simulink model "SistemaCAS_v20"  (R2014a)
settings: Solver=ode3  StartTime=0.0  StopTime=0.009  FixedStep=0.000001  RelTol=1e-3
libraries: simulink x21, dspmathops x10, commchan3 x1
settings Model: Creator=andre  LastModifiedBy=andre
settings DebuggingCC: SolverPrmCheckMsg=none

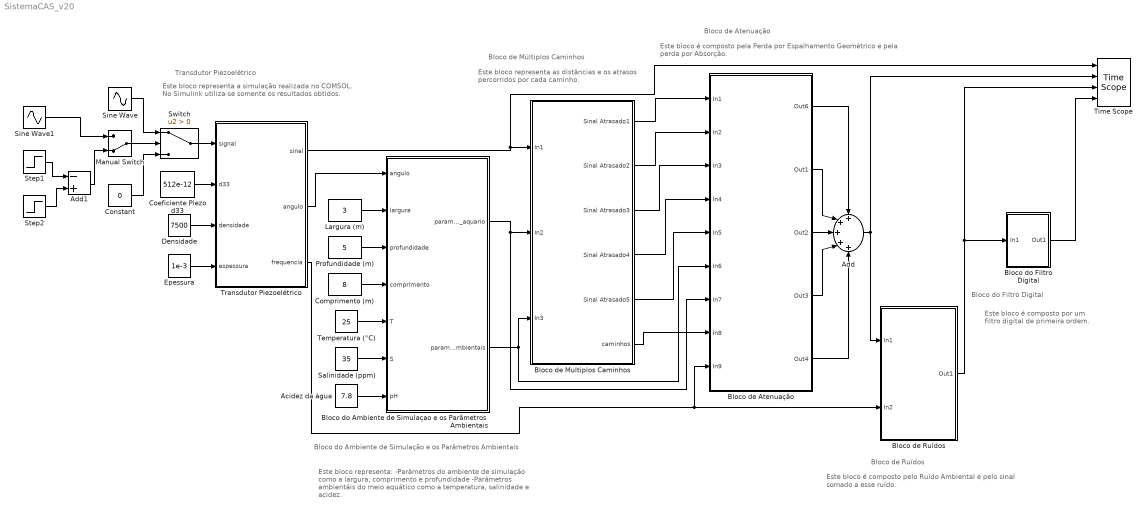
== system SistemaCAS_v20 ==
  note: Este bloco representa a simulação realizada no COMSOL. No Simulink utiliza-se somente os resultados obtidos.
  note: Transdutor Piezoelétrico
  note: Este bloco representa:
      | -Parâmetros do ambiente de simulação como a largura, comprimento e profundidade
      | -Parâmetros ambientáis do meio aquático como a temperatura, salinidade e acidez.
  note: Bloco do Ambiente de Simulação e os Parâmetros Ambientais
  note: Este bloco representa as distâncias e
      | os atrasos percorridos por cada caminho.
  note: Bloco de Múltiplos Caminhos
  note: Este bloco é composto pela Perda por Espalhamento Geométrico e pela perda por Absorção.
  note: Bloco de Atenuação
  note: Este bloco é composto pelo Ruído Ambiental e pelo sinal somado a esse ruído.
  note: Bloco de Ruídos
  note: Este bloco é composto
      | por um filtro digital
      | de primeira ordem.
  note: Bloco do Filtro Digital
  Acidez da água : Constant  Value=7.8
  Add : Sum  Inputs=+++++
  Add1 : Sum  Inputs=-+
  Bloco de Atenuação : Subsystem
  Bloco de Multiplos Caminhos : Subsystem
  Bloco de Ruídos : Subsystem
  Bloco do Ambiente de Simulaçao e os Parâmetros Ambientais : MATLAB Function  TreatAsAtomicUnit=on
  Bloco do Filtro Digital : Subsystem
  Coeficiente Piezo d33 : Constant  Value=512e-12
  Comprimento (m) : Constant  Value=8
  Constant : Constant  Value=0
  Densidade : Constant  Value=7500
  Epessura : Constant  Value=1e-3
  Largura (m) : Constant  Value=3
  Manual Switch : ManualSwitch  CurrentSetting=0
  Profundidade (m) : Constant  Value=5
  Salinidade (ppm) : Constant  Value=35
  Sine Wave : Sin  Amplitude=10  Frequency=19670*(2*pi)  Samples=51  SampleTime=1/1000000
  Sine Wave1 : Sin  Amplitude=10  Frequency=2000*(2*pi)  Samples=100  SampleTime=1/1000000
  Step1 : Step  Time=5*(1/19670)  SampleTime=1/1000000
  Step2 : Step  Time=0  SampleTime=1/1000000
  Switch : Switch  Criteria=u2 > Threshold
  Temperatura (°C) : Constant  Value=25
  Time Scope : TimeScope  NumInputPorts=4  DefaultConfigurationName=spbscopes.TimeScopeBlockCfg
  Transdutor Piezoelétrico : MATLAB Function  TreatAsAtomicUnit=on
  wires:
  Sine Wave/1 -> Switch/1
  Constant/1 -> Switch/3
  Largura (m)/1 -> Bloco do Ambiente de Simulaçao e os Parâmetros Ambientais/2(largura)
  Profundidade (m)/1 -> Bloco do Ambiente de Simulaçao e os Parâmetros Ambientais/3(profundidade)
  Coeficiente Piezo d33/1 -> Transdutor Piezoelétrico/2(d33)
  Densidade/1 -> Transdutor Piezoelétrico/3(densidade)
  Epessura/1 -> Transdutor Piezoelétrico/4(espessura)
  Transdutor Piezoelétrico/2(angulo) -> Bloco do Ambiente de Simulaçao e os Parâmetros Ambientais/1(angulo)
  Bloco do Ambiente de Simulaçao e os Parâmetros Ambientais/1(parametros_aquario) -> Bloco de Atenuação/7(In7), Bloco de Multiplos Caminhos/2(In2)
  Bloco do Ambiente de Simulaçao e os Parâmetros Ambientais/2(parametros_ambientais) -> Bloco de Multiplos Caminhos/3(In3), Bloco de Atenuação/6(In6)
  Switch/1 -> Transdutor Piezoelétrico/1(signal)
  Transdutor Piezoelétrico/3(frequencia) -> Bloco de Ruídos/2(In2), Bloco de Atenuação/9(In9)
  Temperatura (°C)/1 -> Bloco do Ambiente de Simulaçao e os Parâmetros Ambientais/5(T)
  Salinidade (ppm)/1 -> Bloco do Ambiente de Simulaçao e os Parâmetros Ambientais/6(S)
  Acidez da água/1 -> Bloco do Ambiente de Simulaçao e os Parâmetros Ambientais/7(pH)
  Bloco de Multiplos Caminhos/1(Sinal Atrasado1) -> Bloco de Atenuação/1(In1)
  Bloco de Multiplos Caminhos/2(Sinal Atrasado2) -> Bloco de Atenuação/2(In2)
  Bloco de Multiplos Caminhos/3(Sinal Atrasado3) -> Bloco de Atenuação/3(In3)
  Bloco de Multiplos Caminhos/5(Sinal Atrasado5) -> Bloco de Atenuação/5(In5)
  Bloco de Multiplos Caminhos/6(caminhos) -> Bloco de Atenuação/8(In8)
  Bloco de Multiplos Caminhos/4(Sinal Atrasado4) -> Bloco de Atenuação/4(In4)
  Add/1 -> Bloco de Ruídos/1(In1), Time Scope/2
  Bloco de Atenuação/1(Out6) -> Add/1
  Bloco de Atenuação/2(Out1) -> Add/2
  Bloco de Atenuação/3(Out2) -> Add/3
  Bloco de Atenuação/4(Out3) -> Add/4
  Bloco de Atenuação/5(Out4) -> Add/5
  Comprimento (m)/1 -> Bloco do Ambiente de Simulaçao e os Parâmetros Ambientais/4(comprimento)
  Bloco de Ruídos/1(Out1) -> Time Scope/3, Bloco do Filtro Digital/1(In1)
  Step1/1 -> Add1/1
  Step2/1 -> Add1/2
  Manual Switch/1 -> Switch/2
  Sine Wave1/1 -> Manual Switch/1
  Add1/1 -> Manual Switch/2
  Transdutor Piezoelétrico/1(sinal) -> Time Scope/1, Bloco de Multiplos Caminhos/1(In1)
  Bloco do Filtro Digital/1(Out1) -> Time Scope/4

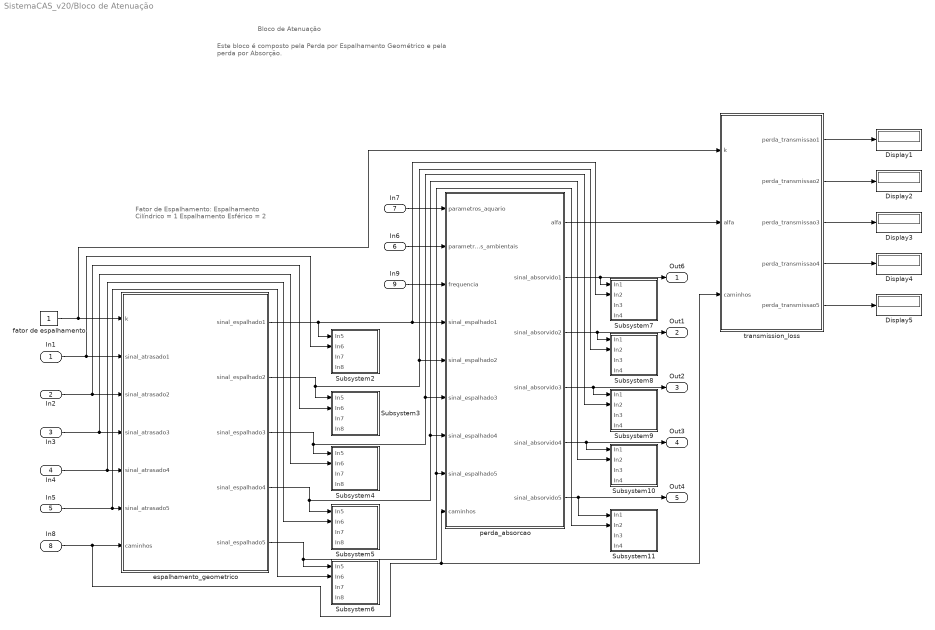
== system SistemaCAS_v20/Bloco de Atenuação ==
  note: Fator de Espalhamento:
      |
      | Espalhamento Cilíndrico = 1
      | Espalhamento Esférico = 2
  note: Este bloco é composto pela Perda por Espalhamento Geométrico e pela perda por Absorção.
  note: Bloco de Atenuação
  In1 : Inport
  In2 : Inport  Port=2
  In3 : Inport  Port=3
  In4 : Inport  Port=4
  In5 : Inport  Port=5
  In6 : Inport  Port=6
  In7 : Inport  Port=7
  In8 : Inport  Port=8
  In9 : Inport  Port=9
  Display{1..5} (5 alike) : Display
      settings: Decimation=2
  Subsystem10 : Subsystem
  Subsystem11 : Subsystem
  Subsystem2 : Subsystem
  Subsystem3 : Subsystem
  Subsystem4 : Subsystem
  Subsystem5 : Subsystem
  Subsystem6 : Subsystem
  Subsystem7 : Subsystem
  Subsystem8 : Subsystem
  Subsystem9 : Subsystem
  espalhamento_geometrico : MATLAB Function  TreatAsAtomicUnit=on
  fator de espalhamento : Constant
  perda_absorcao : MATLAB Function  TreatAsAtomicUnit=on
  transmission_loss : MATLAB Function  TreatAsAtomicUnit=on
  Out6 : Outport
  Out1 : Outport  Port=2
  Out2 : Outport  Port=3
  Out3 : Outport  Port=4
  Out4 : Outport  Port=5
  wires:
  espalhamento_geometrico/1(sinal_espalhado1) -> Subsystem2/1(In5), perda_absorcao/4(sinal_espalhado1), Subsystem7/2(In2)
  In1/1 -> Subsystem2/2(In6), espalhamento_geometrico/2(sinal_atrasado1)
  In3/1 -> Subsystem4/2(In6), espalhamento_geometrico/4(sinal_atrasado3)
  In4/1 -> Subsystem5/2(In6), espalhamento_geometrico/5(sinal_atrasado4)
  fator de espalhamento/1 -> transmission_loss/1(k), espalhamento_geometrico/1(k)
  espalhamento_geometrico/2(sinal_espalhado2) -> Subsystem3/1(In5), perda_absorcao/5(sinal_espalhado2), Subsystem8/2(In2)
  espalhamento_geometrico/5(sinal_espalhado5) -> Subsystem6/1(In5), Subsystem11/2(In2), perda_absorcao/8(sinal_espalhado5)
  espalhamento_geometrico/3(sinal_espalhado3) -> Subsystem4/1(In5), perda_absorcao/6(sinal_espalhado3), Subsystem9/2(In2)
  espalhamento_geometrico/4(sinal_espalhado4) -> Subsystem5/1(In5), perda_absorcao/7(sinal_espalhado4), Subsystem10/2(In2)
  In6/1 -> perda_absorcao/2(parametros_ambientais)
  In7/1 -> perda_absorcao/1(parametros_aquario)
  In9/1 -> perda_absorcao/3(frequencia)
  perda_absorcao/2(sinal_absorvido1) -> Subsystem7/1(In1), Out6/1
  perda_absorcao/5(sinal_absorvido4) -> Out3/1, Subsystem10/1(In1)
  perda_absorcao/6(sinal_absorvido5) -> Out4/1, Subsystem11/1(In1)
  transmission_loss/1(perda_transmissao1) -> Display1/1
  In2/1 -> Subsystem3/2(In6), espalhamento_geometrico/3(sinal_atrasado2)
  perda_absorcao/4(sinal_absorvido3) -> Out2/1, Subsystem9/1(In1)
  perda_absorcao/1(alfa) -> transmission_loss/2(alfa)
  perda_absorcao/3(sinal_absorvido2) -> Out1/1, Subsystem8/1(In1)
  In5/1 -> Subsystem6/2(In6), espalhamento_geometrico/6(sinal_atrasado5)
  In8/1 -> perda_absorcao/9(caminhos), transmission_loss/3(caminhos), espalhamento_geometrico/7(caminhos)
  transmission_loss/2(perda_transmissao2) -> Display2/1
  transmission_loss/3(perda_transmissao3) -> Display3/1
  transmission_loss/4(perda_transmissao4) -> Display4/1
  transmission_loss/5(perda_transmissao5) -> Display5/1

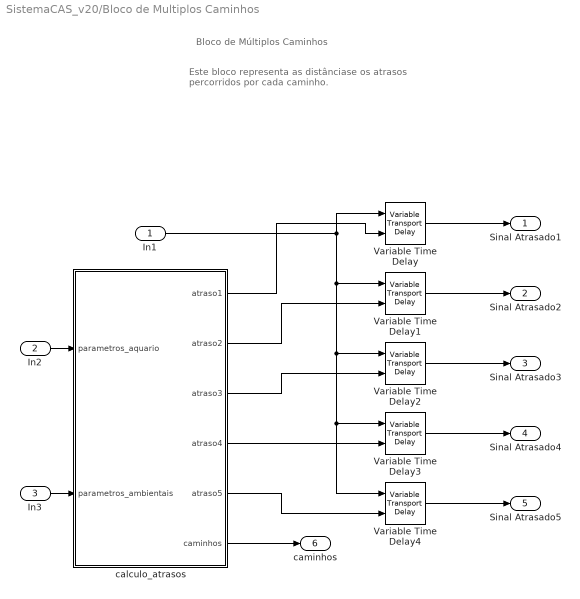
== system SistemaCAS_v20/Bloco de Multiplos Caminhos ==
  note: Este bloco representa as distânciase os atrasos percorridos por cada caminho.
  note: Bloco de Múltiplos Caminhos
  In1 : Inport
  In2 : Inport  Port=2
  In3 : Inport  Port=3
  Variable Time Delay{,1..4} (5 alike) : VariableTransportDelay  MaximumDelay=10
  calculo_atrasos : MATLAB Function  TreatAsAtomicUnit=on
  Sinal Atrasado1 : Outport
  Sinal Atrasado2 : Outport  Port=2
  Sinal Atrasado3 : Outport  Port=3
  Sinal Atrasado4 : Outport  Port=4
  Sinal Atrasado5 : Outport  Port=5
  caminhos : Outport  Port=6
  wires:
  calculo_atrasos/3(atraso3) -> Variable Time Delay2/2
  In2/1 -> calculo_atrasos/1(parametros_aquario)
  In3/1 -> calculo_atrasos/2(parametros_ambientais)
  In1/1 -> Variable Time Delay/1, Variable Time Delay1/1, Variable Time Delay2/1, Variable Time Delay4/1, Variable Time Delay3/1
  calculo_atrasos/1(atraso1) -> Variable Time Delay/2
  Variable Time Delay1/1 -> Sinal Atrasado2/1
  Variable Time Delay3/1 -> Sinal Atrasado4/1
  Variable Time Delay2/1 -> Sinal Atrasado3/1
  calculo_atrasos/6(caminhos) -> caminhos/1
  calculo_atrasos/2(atraso2) -> Variable Time Delay1/2
  calculo_atrasos/4(atraso4) -> Variable Time Delay3/2
  calculo_atrasos/5(atraso5) -> Variable Time Delay4/2
  Variable Time Delay/1 -> Sinal Atrasado1/1
  Variable Time Delay4/1 -> Sinal Atrasado5/1

== system SistemaCAS_v20/Bloco de Ruídos ==
  note: Este bloco é composto pelo Ruído Ambiental e pelo sinal somado a esse ruído.
  note: Bloco de Ruídos
  In1 : Inport
  In2 : Inport  Port=2
  AWGN Channel : commchan3/AWGN Channel  InputProcessing=Columns as channels (frame based)  seed=1  noiseMode=Variance from port  EbNodB=10  EsNodB=10  SNRdB=0  bitsPerSym=1  Ps=1  Tsym=1  variance=1
  To Workspace : ToWorkspace  VariableName=semruido  SaveFormat=Timeseries  SampleTime=-1
  To Workspace1 : ToWorkspace  VariableName=comruido  SaveFormat=Timeseries  SampleTime=-1
  fator de navegação (0-1) : Constant  Value=0
  ruido_ambiente : MATLAB Function  TreatAsAtomicUnit=on
  velocidade do vento (m/s) : Constant  Value=4.17
  Out1 : Outport
  wires:
  In2/1 -> ruido_ambiente/1(frequencia)
  AWGN Channel/1 -> Out1/1, To Workspace1/1
  fator de navegação (0-1)/1 -> ruido_ambiente/2(n)
  velocidade do vento (m/s)/1 -> ruido_ambiente/3(v)
  In1/1 -> To Workspace/1, AWGN Channel/1
  ruido_ambiente/1(ruido_total) -> AWGN Channel/2

== system SistemaCAS_v20/Bloco do Filtro Digital ==
  In1 : Inport
  Transfer Fcn First Order : simulink/Discrete/Transfer Fcn First Order  PoleZ=0.93  ICPrevOutput=0.0  RndMeth=Round  DoSatur=off
  Out1 : Outport
  wires:
  Transfer Fcn First Order/1 -> Out1/1
  In1/1 -> Transfer Fcn First Order/1

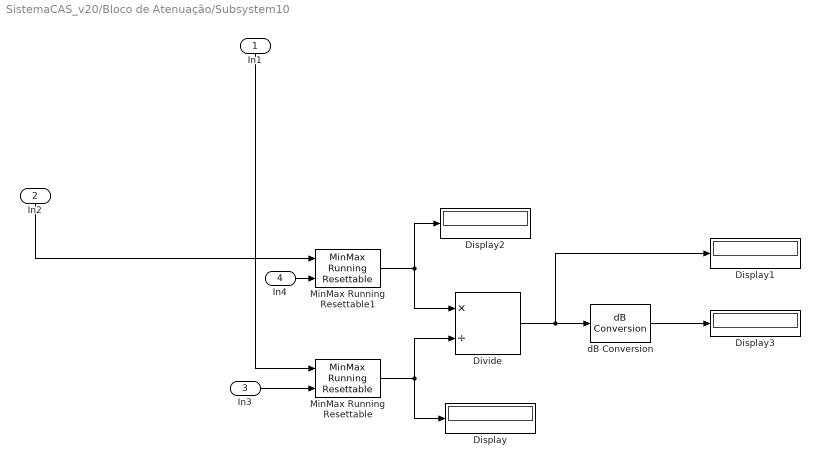
== system SistemaCAS_v20/Bloco de Atenuação/Subsystem10 ==
  In1 : Inport
  In2 : Inport  Port=2
  In3 : Inport  Port=3
  In4 : Inport  Port=4
  Display{,1..3} (4 alike) : Display
      Display1 settings: Decimation=2
      Display3 settings: Decimation=2
  Divide : Product  Inputs=*/
  MinMax Running Resettable : simulink/Math Operations/MinMax Running Resettable  Function=max  vinit=0.0
  MinMax Running Resettable1 : simulink/Math Operations/MinMax Running Resettable  Function=max  vinit=0.0
  dB Conversion : dspmathops/dB Conversion  dBtype=dB  intype=Power  R=1  fuzz=off
  wires:
  In4/1 -> MinMax Running Resettable1/2
  In1/1 -> MinMax Running Resettable/1
  In3/1 -> MinMax Running Resettable/2
  dB Conversion/1 -> Display3/1
  MinMax Running Resettable1/1 -> Display2/1, Divide/1
  MinMax Running Resettable/1 -> Display/1, Divide/2
  Divide/1 -> dB Conversion/1, Display1/1
  In2/1 -> MinMax Running Resettable1/1

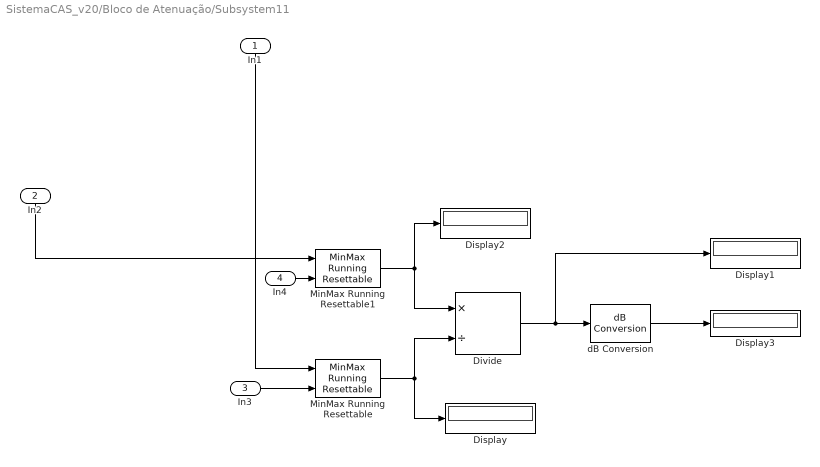
== system SistemaCAS_v20/Bloco de Atenuação/Subsystem11 ==
  In1 : Inport
  In2 : Inport  Port=2
  In3 : Inport  Port=3
  In4 : Inport  Port=4
  Display{,1..3} (4 alike) : Display
      Display1 settings: Decimation=2
      Display3 settings: Decimation=2
  Divide : Product  Inputs=*/
  MinMax Running Resettable : simulink/Math Operations/MinMax Running Resettable  Function=max  vinit=0.0
  MinMax Running Resettable1 : simulink/Math Operations/MinMax Running Resettable  Function=max  vinit=0.0
  dB Conversion : dspmathops/dB Conversion  dBtype=dB  intype=Power  R=1  fuzz=off
  wires:
  In4/1 -> MinMax Running Resettable1/2
  In1/1 -> MinMax Running Resettable/1
  In3/1 -> MinMax Running Resettable/2
  dB Conversion/1 -> Display3/1
  MinMax Running Resettable1/1 -> Display2/1, Divide/1
  MinMax Running Resettable/1 -> Display/1, Divide/2
  Divide/1 -> dB Conversion/1, Display1/1
  In2/1 -> MinMax Running Resettable1/1

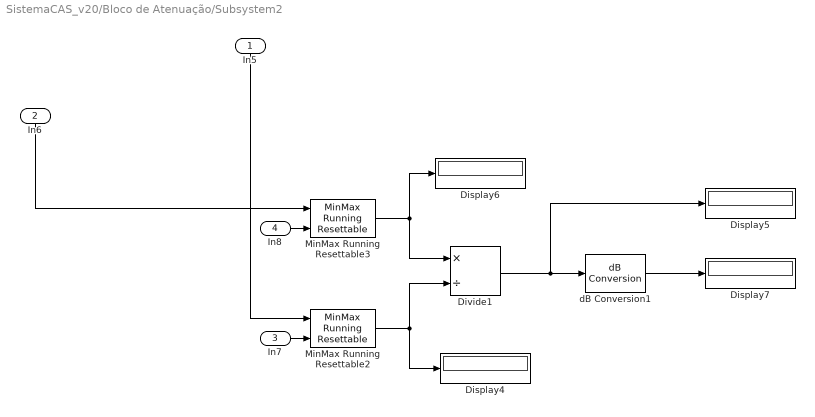
== system SistemaCAS_v20/Bloco de Atenuação/Subsystem2 ==
  In5 : Inport
  In6 : Inport  Port=2
  In7 : Inport  Port=3
  In8 : Inport  Port=4
  Display{4..7} (4 alike) : Display
      Display5 settings: Decimation=2
      Display7 settings: Decimation=2
  Divide1 : Product  Inputs=*/
  MinMax Running Resettable2 : simulink/Math Operations/MinMax Running Resettable  Function=max  vinit=0.0
  MinMax Running Resettable3 : simulink/Math Operations/MinMax Running Resettable  Function=max  vinit=0.0
  dB Conversion1 : dspmathops/dB Conversion  dBtype=dB  intype=Power  R=1  fuzz=off
  wires:
  In8/1 -> MinMax Running Resettable3/2
  In6/1 -> MinMax Running Resettable3/1
  In5/1 -> MinMax Running Resettable2/1
  In7/1 -> MinMax Running Resettable2/2
  dB Conversion1/1 -> Display7/1
  MinMax Running Resettable3/1 -> Display6/1, Divide1/1
  MinMax Running Resettable2/1 -> Display4/1, Divide1/2
  Divide1/1 -> dB Conversion1/1, Display5/1

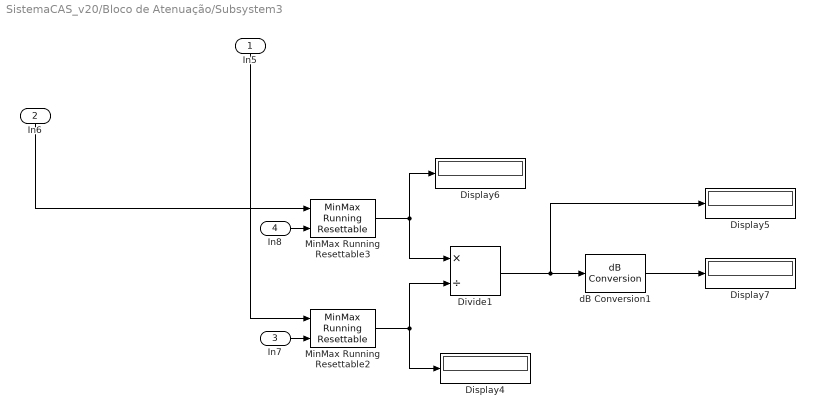
== system SistemaCAS_v20/Bloco de Atenuação/Subsystem3 ==
  In5 : Inport
  In6 : Inport  Port=2
  In7 : Inport  Port=3
  In8 : Inport  Port=4
  Display{4..7} (4 alike) : Display
      Display5 settings: Decimation=2
      Display7 settings: Decimation=2
  Divide1 : Product  Inputs=*/
  MinMax Running Resettable2 : simulink/Math Operations/MinMax Running Resettable  Function=max  vinit=0.0
  MinMax Running Resettable3 : simulink/Math Operations/MinMax Running Resettable  Function=max  vinit=0.0
  dB Conversion1 : dspmathops/dB Conversion  dBtype=dB  intype=Power  R=1  fuzz=off
  wires:
  In8/1 -> MinMax Running Resettable3/2
  In6/1 -> MinMax Running Resettable3/1
  In5/1 -> MinMax Running Resettable2/1
  In7/1 -> MinMax Running Resettable2/2
  dB Conversion1/1 -> Display7/1
  MinMax Running Resettable3/1 -> Display6/1, Divide1/1
  MinMax Running Resettable2/1 -> Display4/1, Divide1/2
  Divide1/1 -> dB Conversion1/1, Display5/1

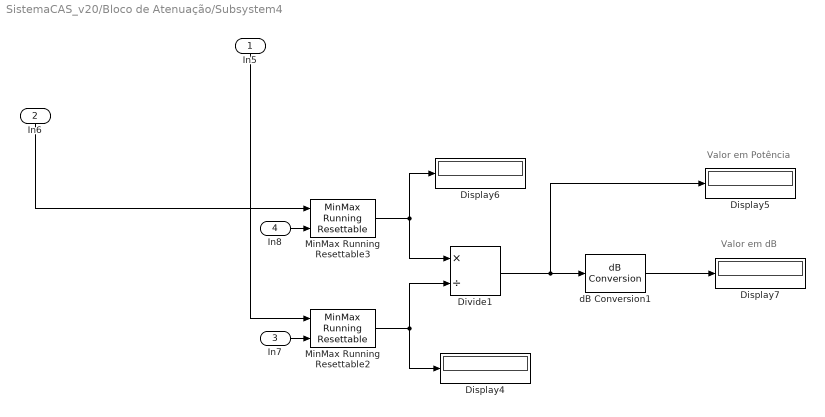
== system SistemaCAS_v20/Bloco de Atenuação/Subsystem4 ==
  note: Valor em dB
  note: Valor em Potência
  In5 : Inport
  In6 : Inport  Port=2
  In7 : Inport  Port=3
  In8 : Inport  Port=4
  Display{4..7} (4 alike) : Display
      Display5 settings: Decimation=2
      Display7 settings: Decimation=2
  Divide1 : Product  Inputs=*/
  MinMax Running Resettable2 : simulink/Math Operations/MinMax Running Resettable  Function=max  vinit=0.0
  MinMax Running Resettable3 : simulink/Math Operations/MinMax Running Resettable  Function=max  vinit=0.0
  dB Conversion1 : dspmathops/dB Conversion  dBtype=dB  intype=Power  R=1  fuzz=off
  wires:
  In8/1 -> MinMax Running Resettable3/2
  In6/1 -> MinMax Running Resettable3/1
  In5/1 -> MinMax Running Resettable2/1
  In7/1 -> MinMax Running Resettable2/2
  dB Conversion1/1 -> Display7/1
  MinMax Running Resettable3/1 -> Display6/1, Divide1/1
  MinMax Running Resettable2/1 -> Display4/1, Divide1/2
  Divide1/1 -> dB Conversion1/1, Display5/1

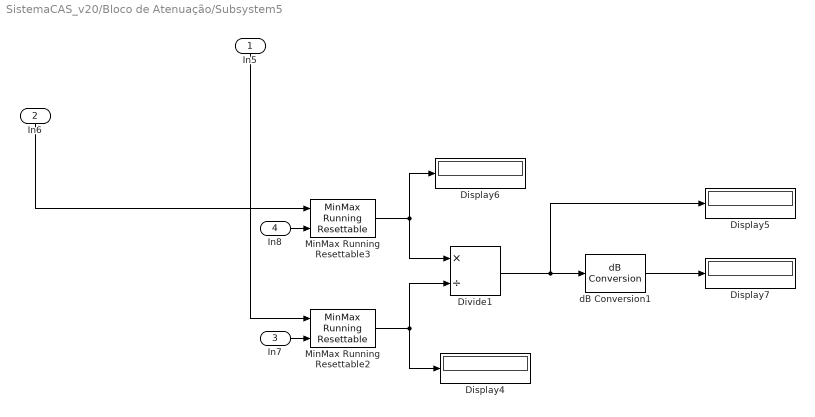
== system SistemaCAS_v20/Bloco de Atenuação/Subsystem5 ==
  In5 : Inport
  In6 : Inport  Port=2
  In7 : Inport  Port=3
  In8 : Inport  Port=4
  Display{4..7} (4 alike) : Display
      Display5 settings: Decimation=2
      Display7 settings: Decimation=2
  Divide1 : Product  Inputs=*/
  MinMax Running Resettable2 : simulink/Math Operations/MinMax Running Resettable  Function=max  vinit=0.0
  MinMax Running Resettable3 : simulink/Math Operations/MinMax Running Resettable  Function=max  vinit=0.0
  dB Conversion1 : dspmathops/dB Conversion  dBtype=dB  intype=Power  R=1  fuzz=off
  wires:
  In8/1 -> MinMax Running Resettable3/2
  In6/1 -> MinMax Running Resettable3/1
  In5/1 -> MinMax Running Resettable2/1
  In7/1 -> MinMax Running Resettable2/2
  dB Conversion1/1 -> Display7/1
  MinMax Running Resettable3/1 -> Display6/1, Divide1/1
  MinMax Running Resettable2/1 -> Display4/1, Divide1/2
  Divide1/1 -> dB Conversion1/1, Display5/1

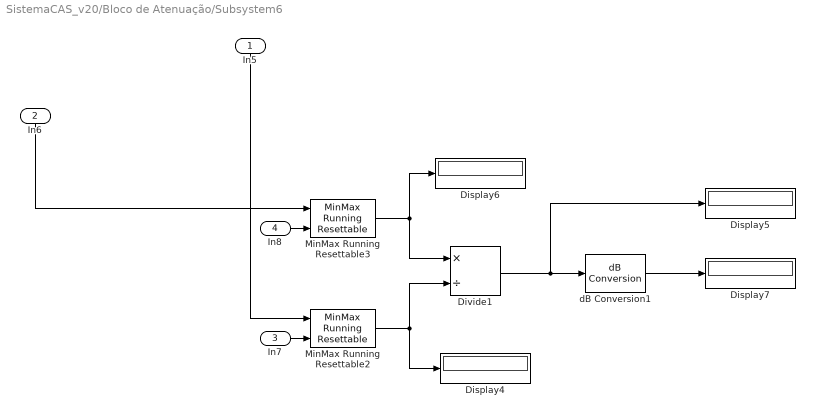
== system SistemaCAS_v20/Bloco de Atenuação/Subsystem6 ==
  In5 : Inport
  In6 : Inport  Port=2
  In7 : Inport  Port=3
  In8 : Inport  Port=4
  Display{4..7} (4 alike) : Display
      Display5 settings: Decimation=2
      Display7 settings: Decimation=2
  Divide1 : Product  Inputs=*/
  MinMax Running Resettable2 : simulink/Math Operations/MinMax Running Resettable  Function=max  vinit=0.0
  MinMax Running Resettable3 : simulink/Math Operations/MinMax Running Resettable  Function=max  vinit=0.0
  dB Conversion1 : dspmathops/dB Conversion  dBtype=dB  intype=Power  R=1  fuzz=off
  wires:
  In8/1 -> MinMax Running Resettable3/2
  In6/1 -> MinMax Running Resettable3/1
  In5/1 -> MinMax Running Resettable2/1
  In7/1 -> MinMax Running Resettable2/2
  dB Conversion1/1 -> Display7/1
  MinMax Running Resettable3/1 -> Display6/1, Divide1/1
  MinMax Running Resettable2/1 -> Display4/1, Divide1/2
  Divide1/1 -> dB Conversion1/1, Display5/1

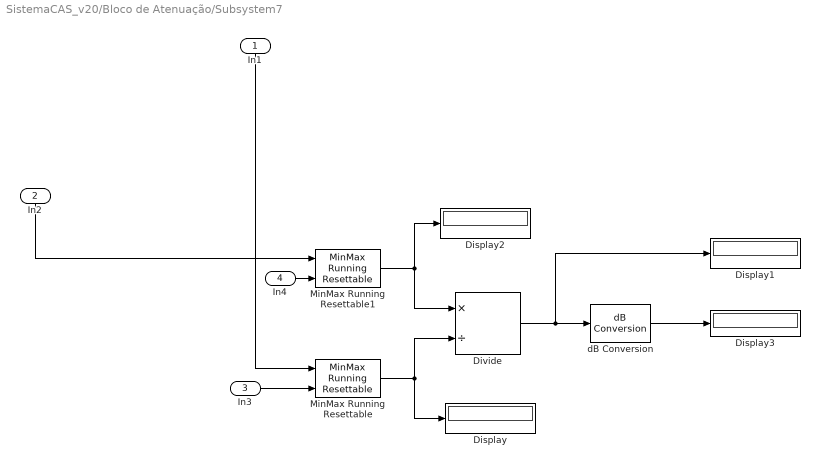
== system SistemaCAS_v20/Bloco de Atenuação/Subsystem7 ==
  In1 : Inport
  In2 : Inport  Port=2
  In3 : Inport  Port=3
  In4 : Inport  Port=4
  Display{,1..3} (4 alike) : Display
      Display1 settings: Decimation=2
      Display3 settings: Decimation=2
  Divide : Product  Inputs=*/
  MinMax Running Resettable : simulink/Math Operations/MinMax Running Resettable  Function=max  vinit=0.0
  MinMax Running Resettable1 : simulink/Math Operations/MinMax Running Resettable  Function=max  vinit=0.0
  dB Conversion : dspmathops/dB Conversion  dBtype=dB  intype=Power  R=1  fuzz=off
  wires:
  In4/1 -> MinMax Running Resettable1/2
  In1/1 -> MinMax Running Resettable/1
  In3/1 -> MinMax Running Resettable/2
  dB Conversion/1 -> Display3/1
  MinMax Running Resettable1/1 -> Display2/1, Divide/1
  MinMax Running Resettable/1 -> Display/1, Divide/2
  Divide/1 -> dB Conversion/1, Display1/1
  In2/1 -> MinMax Running Resettable1/1

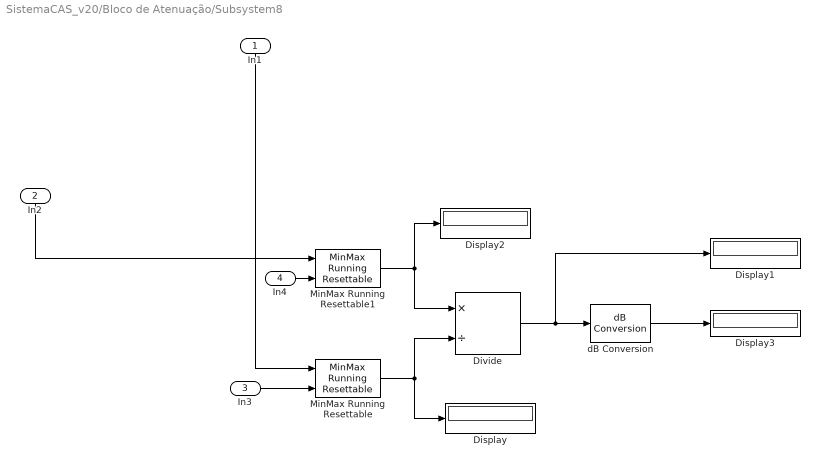
== system SistemaCAS_v20/Bloco de Atenuação/Subsystem8 ==
  In1 : Inport
  In2 : Inport  Port=2
  In3 : Inport  Port=3
  In4 : Inport  Port=4
  Display{,1..3} (4 alike) : Display
      Display1 settings: Decimation=2
      Display3 settings: Decimation=2
  Divide : Product  Inputs=*/
  MinMax Running Resettable : simulink/Math Operations/MinMax Running Resettable  Function=max  vinit=0.0
  MinMax Running Resettable1 : simulink/Math Operations/MinMax Running Resettable  Function=max  vinit=0.0
  dB Conversion : dspmathops/dB Conversion  dBtype=dB  intype=Power  R=1  fuzz=off
  wires:
  In4/1 -> MinMax Running Resettable1/2
  In1/1 -> MinMax Running Resettable/1
  In3/1 -> MinMax Running Resettable/2
  dB Conversion/1 -> Display3/1
  MinMax Running Resettable1/1 -> Display2/1, Divide/1
  MinMax Running Resettable/1 -> Display/1, Divide/2
  Divide/1 -> dB Conversion/1, Display1/1
  In2/1 -> MinMax Running Resettable1/1

== system SistemaCAS_v20/Bloco de Atenuação/Subsystem9 ==
  note: Valor em dB
  note: Valor em Potência
  In1 : Inport
  In2 : Inport  Port=2
  In3 : Inport  Port=3
  In4 : Inport  Port=4
  Display{,1..3} (4 alike) : Display
      Display1 settings: Decimation=2
      Display3 settings: Decimation=2
  Divide : Product  Inputs=*/
  MinMax Running Resettable : simulink/Math Operations/MinMax Running Resettable  Function=max  vinit=0.0
  MinMax Running Resettable1 : simulink/Math Operations/MinMax Running Resettable  Function=max  vinit=0.0
  dB Conversion : dspmathops/dB Conversion  dBtype=dB  intype=Power  R=1  fuzz=off
  wires:
  In4/1 -> MinMax Running Resettable1/2
  In1/1 -> MinMax Running Resettable/1
  In3/1 -> MinMax Running Resettable/2
  dB Conversion/1 -> Display3/1
  MinMax Running Resettable1/1 -> Display2/1, Divide/1
  MinMax Running Resettable/1 -> Display/1, Divide/2
  Divide/1 -> dB Conversion/1, Display1/1
  In2/1 -> MinMax Running Resettable1/1

== matlab function SistemaCAS_v20/Bloco do Ambiente de Simulaçao e os Parâmetros Ambientais ==
  data: angulo input; largura input; profundidade input; comprimento input; parametros_aquario output; parametros_ambientais output; T input; S input; pH input
function [parametros_aquario,parametros_ambientais] = ambiente_simulado(angulo,largura,profundidade,comprimento,T,S,pH)
% consideraçoes para os parâmetros do aquário
% 1. emissor e receptor estão alinhados ( largura(x) e profundidade(z)
% iguais, só muda o comprimento (y)
% 2. o comprimento do aquario (L) é ideal para acontecer uma reflexão completa
% com o angulo de diretividade (que é o maior angulo possível do lóbulo 
% principal utilizando o transdutor piezoeletrico escolhido)
% 3. para facilitar os cálculos de do comprimento ideal, utilizamos largura
% igual profundidade (D = W)

% considerações sobre a simulação
% 1. serão considerados somente os caminhos do angulo de diretividade e o
% caminho direto (5 caminhos: um direto, dois que refletem nas laterais, e
% dois que refletem na superfície e o fundo
% 2. a reflexão será considerada reflexão completa com um eco (sem perdas 
% de energia ou refraçao)

%-------------------------------------------------------------------------
%Parâmetros do Aquário definidos anteriormente
%-------------------------------------------------------------------------
W = largura;                   % largura (eixo x)
D = profundidade;              % profundidade do aquário (eixo z) 
%L = W/sin(angulo/2)           % comprimento do aquário calculado utilizando o angulo de diretividade (eixo y)
L = comprimento;               % L é a distancia ideal para acontecer uma reflexão completa

parametros_aquario = [W,L,D];

%-------------------------------------------------------------------------
% Valores dos parâmetros do meio subaquático 
%-------------------------------------------------------------------------
%T = 30;                 % Temperatura (°C)
%S = 1;                  % Salinidade (ppt)
%pH = 7.2;               % acidêz da água - pH (potencial hidrogeniônico)
parametros_ambientais = [T, S, pH];

== matlab function SistemaCAS_v20/Bloco de Multiplos Caminhos/calculo_atrasos ==
  data: atraso1 output; atraso2 output; atraso3 output; atraso4 output; atraso5 output; parametros_aquario input; parametros_ambientais input; caminhos output
function [atraso1,atraso2,atraso3,atraso4,atraso5,caminhos] = calculo_atrasos(parametros_aquario,parametros_ambientais)
%Definir as distâncias de cada caminho do multipath;
%Definir a profundidade media para cada caminho do multipath;
%Equação para Velocidade do som na água; 
%Atrasar o sinal de cada caminho do multipath;

%-------------------------------------------------------------------------
% Parametros do aquário e do ambiente que serao utilizados no código 
%-------------------------------------------------------------------------

W = parametros_aquario(1);      %W é a largura do aquário
L = parametros_aquario(2);      %L é comprimento do aquário
D = parametros_aquario(3);      %D é a profundidade do aquário

T = parametros_ambientais(1);   %T é a temperatura da água;
S = parametros_ambientais(2);   %S é a salinidade da água;
pH = parametros_ambientais(3);  %pH é acidez da água;

%-------------------------------------------------------------------------
% Definindo as distâncias em kilometros de cada caminho do multipath entre o 
% emissor e o receptor
%-------------------------------------------------------------------------
% distancias(1) = caminho refletido na superfície
% distancias(2) = caminho refletido na lateral de trás
% distancias(3) = caminho direto
% distancias(4) = caminho refletido na lateral da frente
% distancias(5) = caminho refletido no fundo
%-------------------------------------------------------------------------

distancias = [0 0 0 0 0];        %em metros
distancias(1) = sqrt(D^2 + L^2);
distancias(2) = sqrt(W^2 + L^2);
distancias(3) = L;               %L é comprimento do aquário
distancias(4) = sqrt(W^2 + L^2);
distancias(5) = sqrt(D^2 + L^2);

%-------------------------------------------------------------------------
%Definindo a profundidade média(Dm) em metros para cada caminho, considerando que os
%transdutores estão localizados na metade do aquário e alinhados entre si.
%-------------------------------------------------------------------------

Dm = [0 0 0 0 0];               % em metros
Dm(1) = mean([D/2,0]);
Dm(2) = D/2;
Dm(3) = D/2;
Dm(4) = D/2;
Dm(5) = mean([D,D/2]);

%-------------------------------------------------------------------------
%Equação que define a Velocidade do som na água em (m/s)
%-------------------------------------------------------------------------

C = [0 0 0 0 0];
for i = 1:5 %5 caminhos
    C(i) = 1448.96 + 4.591*T - 5.304*(10^(-2))*(T^(2))...
        + 2.374*(10^(-4))*(T^(3)) + 1.340*(S-35) + 1.630*(10^(-2))*Dm(i)...
        + 1.675*(10^(-7))*(Dm(i)^(2)) - 1.025*(10^(-2))*T*(S-35)...
        - 7.139*(10^(-13))*T*(Dm(i)^(3));
end

%-------------------------------------------------------------------------
% Definindo os atrasos em segundos para cada caminho do multipath.
% O atraso é descoberto através da divisão da distância em metros 
% pela velocidade do som na agua em metros/segundos.
%-------------------------------------------------------------------------

atraso1 = distancias(1)/C(1);
atraso2 = distancias(2)/C(2);
atraso3 = distancias(3)/C(3);  
atraso4 = distancias(4)/C(4);
atraso5 = distancias(5)/C(5);

caminhos = distancias;

%a = 10^8;
%atraso1 = atraso1*a;
%atraso2 = atraso2*a;
%atraso3 = atraso3*a;
%atraso4 = atraso4*a;
%atraso5 = atraso5*a;

== matlab function SistemaCAS_v20/Bloco de Atenuação/perda_absorcao ==
  data: alfa output; parametros_aquario input; parametros_ambientais input; frequencia input; sinal_espalhado1 input; sinal_espalhado2 input; sinal_espalhado3 input; sinal_espalhado4 input; sinal_espalhado5 input; caminhos input; sinal_absorvido1 output; sinal_absorvido2 output; sinal_absorvido3 output; sinal_absorvido4 output; sinal_absorvido5 output
function [alfa,sinal_absorvido1,sinal_absorvido2,sinal_absorvido3,sinal_absorvido4,...
    sinal_absorvido5]  = perda_absorcao(parametros_aquario,parametros_ambientais,...
    frequencia,sinal_espalhado1,sinal_espalhado2,sinal_espalhado3,sinal_espalhado4,...
    sinal_espalhado5,caminhos)
% Calcular o coeficeinte de absorção (alfa)
% Calcular a perda por absorção

% Parâmetros Ambientais
T = parametros_ambientais(1);       % Temperatura da água
S = parametros_ambientais(2);       % Salinidade da água do mar do litoral brasileiro (1 milligram/liter [mg/L] = 1,000000002 part/million [ppm])
pH = parametros_ambientais(3);      % Acidez da água

% Parâmetro da Geometria do Aquário
D = parametros_aquario(3);          % Profundidade em m

%c = 1412 + 3.21*T + 1.19*S + 0.0167*D;  % velocidade do som em metros/segundos

%Valores dos parâmetros Para o primeiro Coeficiente de Absorção(alfa)  
f1 = 0.78 * sqrt(S/35) * (exp(T/26));    % Ácido Bórico
f2 = 42 * (exp(T/17));                   % Sulfato de Magnésio

%-------------------------------------------------------------------------
%Equação que define Coeficiente de Absorção(alfa) para a profundidade 
%média (Dm) em cada caminho.
%-------------------------------------------------------------------------
frequencia = frequencia * 0.001;        %kHz
D = D * 0.001;                          %km

%Profundidade média do aquário
Dm = [0 0 0 0 0];
Dm(1) = mean([D/2,0]);
Dm(2) = D/2;
Dm(3) = D/2;
Dm(4) = D/2;
Dm(5) = mean([D,D/2]);

alfa = [0 0 0 0 0];
for i = 1:5         %5 caminhos em profundidades diferentes
    alfa(i) = ((0.106 * (f1 * frequencia^2) * exp((pH - 8) / 0.56)) / ...
        (f1^2 + frequencia^2)) + ((0.52 * (1 + (T / 43)) * (S / 35) * ...
        (f2 * frequencia^2) * exp(-(Dm(i) / 6))) / (f2^2 + frequencia^2)) + ...
        (0.00049 * (frequencia^2) * (exp(-(T/27 + Dm(i)/17))));
end

%a = 10*log10(alfa);

%--------------------------------------------------------------------------
% Perda_absorção = 10log(alfa)*caminhos(km)                 (dB/km) 
%--------------------------------------------------------------------------
perda_absorcao1 = 10*log10(alfa(1))*caminhos(1)*0.001;
perda_absorcao2 = 10*log10(alfa(2))*caminhos(2)*0.001;
perda_absorcao3 = 10*log10(alfa(3))*caminhos(3)*0.001;
perda_absorcao4 = 10*log10(alfa(4))*caminhos(4)*0.001;
perda_absorcao5 = 10*log10(alfa(5))*caminhos(5)*0.001;

%-------------------------------------------------------------------------
% Equação para a absorvição do sinal utilizando a razao normal de ganho
% em que G=(Pout/Pin)<1
% in = sinal_espalhado*10^(atenuacao/10) 
%-------------------------------------------------------------------------
sinal_absorvido1 = sinal_espalhado1.*(10^(-perda_absorcao1/10));
sinal_absorvido2 = sinal_espalhado2.*(10^(-perda_absorcao2/10));
sinal_absorvido3 = sinal_espalhado3.*(10^(-perda_absorcao3/10));
sinal_absorvido4 = sinal_espalhado4.*(10^(-perda_absorcao4/10));
sinal_absorvido5 = sinal_espalhado5.*(10^(-perda_absorcao5/10));

== matlab function SistemaCAS_v20/Bloco de Atenuação/espalhamento_geometrico ==
  data: k input; sinal_atrasado1 input; sinal_atrasado2 input; sinal_atrasado3 input; sinal_atrasado4 input; sinal_atrasado5 input; sinal_espalhado1 output; sinal_espalhado2 output; sinal_espalhado3 output; sinal_espalhado4 output; sinal_espalhado5 output; caminhos input
function [sinal_espalhado1,sinal_espalhado2,sinal_espalhado3,sinal_espalhado4,...
    sinal_espalhado5] = espalhamento_geometrico(k,sinal_atrasado1,...
    sinal_atrasado2,sinal_atrasado3,sinal_atrasado4,sinal_atrasado5,caminhos)
%a perda por espalhamento geométrico é calculado a partir da equação da
%dissertação:   perda_espalhamento = k * 10log(r); 
%   k = fator de espalhamento
%   caminhos = distância em metros que o sinal percorre ao longo da propagação

%-------------------------------------------------------------------------
%Equação para cálculo da perda por espalhamento geométrico (Spreading Loss)
%-------------------------------------------------------------------------
perda_espalhamento1 = k*10*log10(caminhos(1));
perda_espalhamento2 = k*10*log10(caminhos(2));
perda_espalhamento3 = k*10*log10(caminhos(3));
perda_espalhamento4 = k*10*log10(caminhos(4));
perda_espalhamento5 = k*10*log10(caminhos(5));

%-------------------------------------------------------------------------
% Equação para o espalhamento do sinal utilizando a razao normal de ganho
% em que G=(Pout/Pin)<1
% in = sinal_atrasado*10^(perda_espalhamento/10)
%-------------------------------------------------------------------------
sinal_espalhado1 = sinal_atrasado1.*(10^(-perda_espalhamento1/10));
sinal_espalhado2 = sinal_atrasado2.*(10^(-perda_espalhamento2/10));
sinal_espalhado3 = sinal_atrasado3.*(10^(-perda_espalhamento3/10));
sinal_espalhado4 = sinal_atrasado4.*(10^(-perda_espalhamento4/10));
sinal_espalhado5 = sinal_atrasado5.*(10^(-perda_espalhamento5/10));

== matlab function SistemaCAS_v20/Transdutor Piezoelétrico ==
  data: signal input; d33 input; sinal output; densidade input; espessura input; angulo output; frequencia output
function [sinal,angulo,frequencia] = projetor(signal,d33,densidade,espessura)
%-------------------------------------------------------------------------
% Sinal 
%-------------------------------------------------------------------------
sinal=signal;

%-------------------------------------------------------------------------
% Ângulo de diretividade do transdutor calculado no COMSOL (rad)
%(ex.: 60º = pi/3 rad)
angulo = 0.890852426;       %rad
%-------------------------------------------------------------------------
% angulo1 = 0.859373542;	%49.24° com ganho de 13449.18484
% angulo2 = 0.890852426;	%51.04°	com ganho de 13150.20387
% angulo3 = 0.92233131;     %52.85°	com ganho de 11640.72903
% angulo4 = 0.790119996;	%45.27°	com ganho de 10759.71489
% angulo5 = 0.022035219;	%1.26°	com ganho de 10755.78133
% angulo6 = 0.015739442;	%0.90°	com ganho de 10755.46206
% angulo7 = 0.009443665;	%0.54°	com ganho de 10744.9723
% angulo8 = 0.003147888;	%0.18°	com ganho de 10735.05893 

%-------------------------------------------------------------------------
% Frequência do Sinal (Hz)
%-------------------------------------------------------------------------
frequencia = 19670;

== matlab function SistemaCAS_v20/Bloco de Ruídos/ruido_ambiente ==
  data: ruido_total output; frequencia input; n input; v input
function ruido_total = ruido_ambiente(frequencia,n,v)
%-------------------------------------------------------------------------
%Parâmetros de entrada do ruido ambiental
%-------------------------------------------------------------------------
f = frequencia;                 % frequência (kHz); 
%n = inserido como constante    % fator de navegaçao(entre 0 - 1);
%v = inserido como constante    % velocidade do vento (m/s); 

%-------------------------------------------------------------------------
%Ruído de Turbulência definido pela Equação (dB)(influencia frequencias < 10 Hz) 
%-------------------------------------------------------------------------
Nt = (10^((17-30*log10(f))/10));

%-------------------------------------------------------------------------
%Ruído de Navegações definido pela Equação (dB)(influencia frequencias entre 10 - 100 Hz)
%-------------------------------------------------------------------------
Ns = (10^((40+(20*(n-0.5))+(26*log10(f))-(60*log10(f+0.03)))/10));

%-------------------------------------------------------------------------
%Ruído das Ondas definido pela Equação (dB)(influencia freuencias entre 100 Hz - 100 kHz)
%-------------------------------------------------------------------------
%Explicar no texto que a influencia do ruído é muito pequena para o nosso cenário e o porque
%Colocar a figura do artigo [on the relationship...]

%Ruído de Agitação de Superfície (Surface Agitation Noise)

Nw = (10^((50+(7.5*(v^(1/2)))+(20*log10(f))-(40*log10(f+0.4)))/10));

%-------------------------------------------------------------------------
%Ruído Térmico definido pela Equação (dB)(influencia frequencias > 100 kHz)
%-------------------------------------------------------------------------
Nth = (10^((-15+20*log10(f))/10));

%-------------------------------------------------------------------------
%Ruído Total definido pelo somatório de todos os ruidos ambientais (dB)
%-------------------------------------------------------------------------
%ruido_total = 10*log10(Nt + Ns + Nw + Nth);
%ruido_total = 10*log10(Nw);

ruido_total = Nw;

== matlab function SistemaCAS_v20/Bloco de Atenuação/transmission_loss ==
  data: k input; alfa input; perda_transmissao1 output; caminhos input; perda_transmissao2 output; perda_transmissao3 output; perda_transmissao4 output; perda_transmissao5 output
function [perda_transmissao1,perda_transmissao2,perda_transmissao3,...
    perda_transmissao4,perda_transmissao5] = transmission_loss(k,alfa,...
    caminhos)
%--------------------------------------------------------------------------
% r = caminho = distância (m)
% alfa = coeficiente de absorção (dB/km)

%A equação que define a perda de transmissão para ambientes de aguas rasas
%é dada pela expressão:

%TL = SL + AL (dB)
%perda_transmissao = perda_espalhamento + perda_absorcao

perda_transmissao1 = 10*log10(10^((k*10*log10(caminhos(1)))/10) + 10^((10*log10(alfa(1))*caminhos(1)*0.001)/10));
perda_transmissao2 = 10*log10(10^((k*10*log10(caminhos(2)))/10) + 10^((10*log10(alfa(2))*caminhos(2)*0.001)/10));
perda_transmissao3 = 10*log10(10^((k*10*log10(caminhos(3)))/10) + 10^((10*log10(alfa(3))*caminhos(3)*0.001)/10));
perda_transmissao4 = 10*log10(10^((k*10*log10(caminhos(4)))/10) + 10^((10*log10(alfa(4))*caminhos(4)*0.001)/10));
perda_transmissao5 = 10*log10(10^((k*10*log10(caminhos(5)))/10) + 10^((10*log10(alfa(5))*caminhos(5)*0.001)/10));

%perda_transmissao = (perda_transmissao1+perda_transmissao2+perda_transmissao3...
   % +perda_transmissao4+perda_transmissao5)/5
